simulink model "autotun2_1stor_mod"  (R2025b)
settings: Solver=ode4  StartTime=0.0  StopTime=50  FixedStep=Tm  RelTol=1e-3
values from neighbouring files (symbols this model uses):
  Delay = 0.005    [twodo_par1.m]
  Tm = St    (= 0.001)    [twodo_par1.m]
libraries: fuzblock x2
settings Model: ExtModeTrigMode=oneshot  ExtModeArmWhenConnect=off  Creator=rel  LastModifiedBy=labrobm
settings DataIOCC: SaveFormat=Array  SignalLoggingSaveFormat=ModelDataLogs  ReturnWorkspaceOutputs=off  SignalLoggingName=sigsOut
settings OptimizationCC: BlockReduction=off  BooleanDataType=off
settings DebuggingCC: SaveWithParameterizedLinksMsg=none  UnderspecifiedInitializationDetection=Classic  MergeDetectMultiDrivingBlocksExec=none  SignalResolutionControl=TryResolveAllWithWarning  MultiTaskDSMMsg=warning  MultiTaskCondExecSysMsg=none  UnconnectedInputMsg=warning  UnconnectedOutputMsg=warning  UnconnectedLineMsg=warning
settings HardwareCC: ProdBitPerPointer=32.0  ProdBitPerSizeT=32.0  ProdBitPerPtrDiffT=32.0  ProdLargestAtomicFloat=None  ProdIntDivRoundTo=Undefined  ProdEndianess=Unspecified  ProdWordSize=32.0  ProdHWDeviceType=32-bit Generic  TargetUnknown=on
settings ModelReferenceCC: PropagateSignalLabelsOutOfModel=off
settings GRTTargetCC: CombineOutputUpdateFcns=off  GRTInterface=on
settings ConfigComp: CovMetricSettings=dw  CovSaveCumulativeToWorkspaceVar=on  CovSaveSingleToWorkspaceVar=on

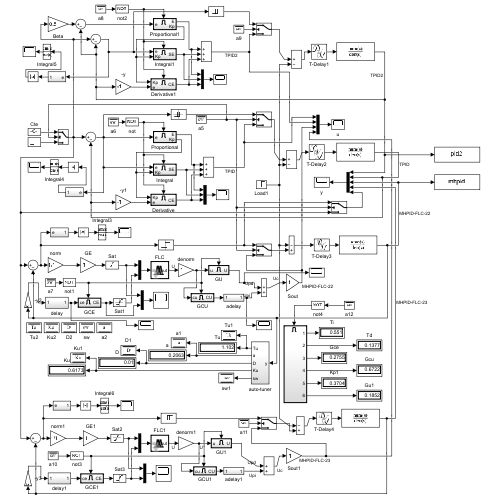
[thumbnail: Simulink's stored preview of the top-level diagram]
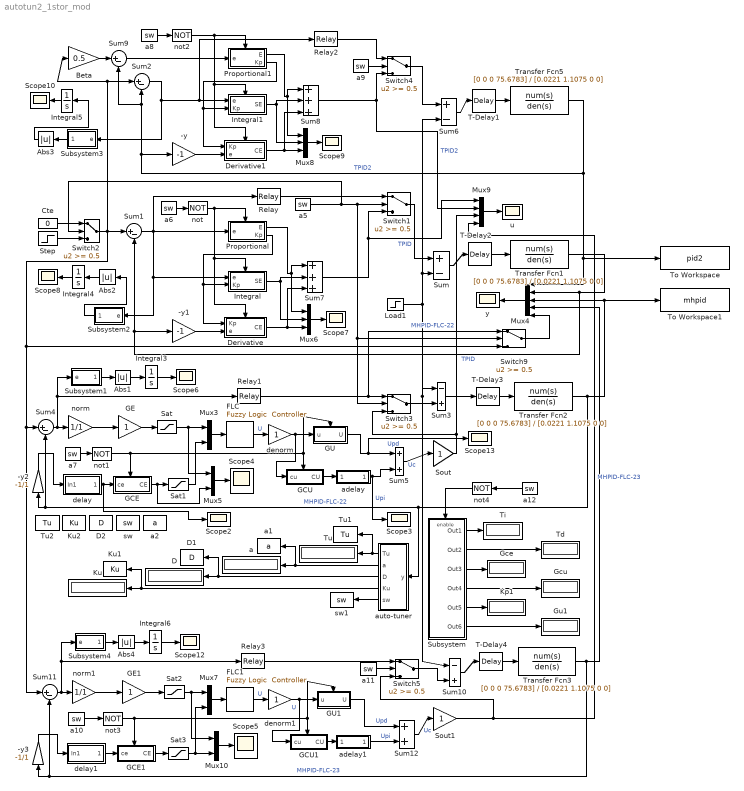
== system autotun2_1stor_mod ==
  -y : Gain  Gain=-1  SaturateOnIntegerOverflow=on  OutDataTypeStr=Inherit: Same as input  ParamDataTypeStr=Inherit: Same as input
  -y1 : Gain  Gain=-1  SaturateOnIntegerOverflow=on  OutDataTypeStr=Inherit: Same as input  ParamDataTypeStr=Inherit: Same as input
  -y2 : Gain  Gain=-1/1  SaturateOnIntegerOverflow=on  OutDataTypeStr=Inherit: Same as input  ParamDataTypeStr=Inherit: Same as input
  -y3 : Gain  Gain=-1/1  SaturateOnIntegerOverflow=on  OutDataTypeStr=Inherit: Same as input  ParamDataTypeStr=Inherit: Same as input
  Abs{1..4} (4 alike) : Abs
  Beta : Gain  Gain=0.5  SaturateOnIntegerOverflow=on  OutDataTypeStr=Inherit: Same as input  ParamDataTypeStr=Inherit: Same as input
  Cte : Constant  Value=0
  D : Display
  D1 : DataStoreWrite  DataStoreName=D  IndexOptions=Index vector (dialog)  Indices=1  OutputSizes=1
  D2 : DataStoreMemory  DataStoreName=D  ShowAdditionalParam=off
  Derivative : Subsystem  TreatAsAtomicUnit=on
  Derivative1 : Subsystem  TreatAsAtomicUnit=on
  FLC : fuzblock/Fuzzy Logic  Controller  FIS=stfc22  OutputSampleNumber=101  DataType=double  UseLookupTable=off  NumBreakpoints=10  FuzzifiedInputs=off  RuleFiringStrengths=off  RuleOutputs=off  AggregatedOutputs=off  SimulateUsing=Interpreted execution  OutOfRangeInputValueMessage=warning  NoRuleFiredMessage=warning  EmptyOutputFuzzySetMessage=warning
  FLC1 : fuzblock/Fuzzy Logic  Controller  FIS=stfc23  OutputSampleNumber=101  DataType=double  UseLookupTable=off  NumBreakpoints=10  FuzzifiedInputs=off  RuleFiringStrengths=off  RuleOutputs=off  AggregatedOutputs=off  SimulateUsing=Interpreted execution  OutOfRangeInputValueMessage=warning  NoRuleFiredMessage=warning  EmptyOutputFuzzySetMessage=warning
  GCE : Subsystem  TreatAsAtomicUnit=on
  GCE1 : Subsystem  TreatAsAtomicUnit=on
  GCU : Subsystem  TreatAsAtomicUnit=on
  GCU1 : Subsystem  TreatAsAtomicUnit=on
  GE : Gain  SaturateOnIntegerOverflow=on  OutDataTypeStr=Inherit: Same as input  ParamDataTypeStr=Inherit: Same as input
  GE1 : Gain  SaturateOnIntegerOverflow=on  OutDataTypeStr=Inherit: Same as input  ParamDataTypeStr=Inherit: Same as input
  GU : Subsystem  TreatAsAtomicUnit=on
  GU1 : Subsystem  TreatAsAtomicUnit=on
  Gce : Display
  Gcu : Display
  Gu1 : Display
  Integral : Subsystem  TreatAsAtomicUnit=on
  Integral1 : Subsystem  TreatAsAtomicUnit=on
  Integral{3..6} (4 alike) : TransferFcn  Denominator=[1 0]
  Kp1 : Display
  Ku : Display
  Ku1 : DataStoreWrite  DataStoreName=Ku  IndexOptions=Index vector (dialog)  Indices=1  OutputSizes=1
  Ku2 : DataStoreMemory  DataStoreName=Ku  ShowAdditionalParam=off
  Load1 : Step  Time=40  SampleTime=0
  Mux{3,5,7,10} (4 alike) : Mux  Inputs=2
  Mux4 : Mux  Inputs=5
  Mux6 : Mux  Inputs=3
  Mux8 : Mux  Inputs=3
  Mux9 : Mux
  Proportional : Subsystem  TreatAsAtomicUnit=on
  Proportional1 : Subsystem  TreatAsAtomicUnit=on
  Relay{,1..3} (4 alike) : Relay  OnOutputValue=0.1  OffOutputValue=-0.1
  Sat{,1..3} (4 alike) : Saturate  UpperLimit=1  LowerLimit=-1
  Scope{2..10,12..13} (11 alike) : Scope
      Scope10 settings: TimeSpan=40  ActiveDisplayYMinimum=0  ActiveDisplayYMaximum=1.5
      Scope12 settings: TimeSpan=40  ActiveDisplayYMinimum=0  ActiveDisplayYMaximum=1.73154
      Scope13 settings: TimeSpan=50  ActiveDisplayYMinimum=-0.01  ActiveDisplayYMaximum=0.05
      Scope2 settings: TimeSpan=50  ActiveDisplayYMinimum=-0.02  ActiveDisplayYMaximum=0.01
      Scope3 settings: TimeSpan=50  ActiveDisplayYMinimum=-0.90801012374905665  ActiveDisplayYMaximum=1.7443936739549131
      Scope4 settings: TimeSpan=50  ActiveDisplayYMinimum=-1  ActiveDisplayYMaximum=1
      Scope5 settings: TimeSpan=40  ActiveDisplayYMinimum=-1  ActiveDisplayYMaximum=1
      Scope6 settings: TimeSpan=40  ActiveDisplayYMinimum=0  ActiveDisplayYMaximum=2
      Scope7 settings: TimeSpan=40  ActiveDisplayYMinimum=-50  ActiveDisplayYMaximum=150
      Scope8 settings: TimeSpan=40  ActiveDisplayYMinimum=0  ActiveDisplayYMaximum=1.77181
      Scope9 settings: TimeSpan=50  ActiveDisplayYMinimum=-2.71141  ActiveDisplayYMaximum=4
  Sout : Gain  SaturateOnIntegerOverflow=on  OutDataTypeStr=Inherit: Same as input  ParamDataTypeStr=Inherit: Same as input
  Sout1 : Gain  SaturateOnIntegerOverflow=on  OutDataTypeStr=Inherit: Same as input  ParamDataTypeStr=Inherit: Same as input
  Step : Step  Time=30  SampleTime=0
  Subsystem : Subsystem  TreatAsAtomicUnit=on
  Subsystem1 : Subsystem
  Subsystem2 : Subsystem
  Subsystem3 : Subsystem
  Subsystem4 : Subsystem
  Sum{,1..2,4,6,9,11} (7 alike) : Sum  Inputs=|+-  InputSameDT=on  SaturateOnIntegerOverflow=on  OutDataTypeStr=Inherit: Same as first input
  Sum10 : Sum  Inputs=|-+  InputSameDT=on  SaturateOnIntegerOverflow=on  OutDataTypeStr=Inherit: Same as first input
  Sum12 : Sum  Inputs=|++  InputSameDT=on  SaturateOnIntegerOverflow=on  OutDataTypeStr=Inherit: Same as first input
  Sum3 : Sum  Inputs=|-+  InputSameDT=on  SaturateOnIntegerOverflow=on  OutDataTypeStr=Inherit: Same as first input
  Sum5 : Sum  Inputs=|++  InputSameDT=on  SaturateOnIntegerOverflow=on  OutDataTypeStr=Inherit: Same as first input
  Sum7 : Sum  Inputs=|+++  InputSameDT=on  SaturateOnIntegerOverflow=on  OutDataTypeStr=Inherit: Same as first input
  Sum8 : Sum  Inputs=|+++  InputSameDT=on  SaturateOnIntegerOverflow=on  OutDataTypeStr=Inherit: Same as first input
  Switch{1..5,9} (6 alike) : Switch  Threshold=0.5
  T-Delay{1..4} (4 alike) : TransportDelay  DelayTime=Delay
  Td : Display
  Ti : Display
  To Workspace : ToWorkspace  VariableName=pid2  SaveFormat=Timeseries  SampleTime=-1
  To Workspace1 : ToWorkspace  VariableName=mhpid  SaveFormat=Timeseries  SampleTime=-1
  Transfer Fcn{1..3,5} (4 alike) : TransferFcn  Numerator=[0 0 0 75.6783]  Denominator=[0.0221 1.1075 0 0]
  Tu : Display
  Tu1 : DataStoreWrite  DataStoreName=Tu  IndexOptions=Index vector (dialog)  Indices=1  OutputSizes=1
  Tu2 : DataStoreMemory  DataStoreName=Tu  InitialValue=1  ShowAdditionalParam=off
  a : Display
  a1 : DataStoreWrite  DataStoreName=a  IndexOptions=Index vector (dialog)  Indices=1  OutputSizes=1
  a{5..12} (8 alike) : DataStoreRead  DataStoreName=sw  SampleTime=0  IndexOptions=Index vector (dialog)  Indices=1  OutputSizes=1
  a2 : DataStoreMemory  DataStoreName=a  ShowAdditionalParam=off
  adelay : Subsystem
  adelay1 : Subsystem
  auto-tuner : Subsystem
  delay : Subsystem
  delay1 : Subsystem
  denorm : Gain  SaturateOnIntegerOverflow=on  OutDataTypeStr=Inherit: Same as input  ParamDataTypeStr=Inherit: Same as input
  denorm1 : Gain  SaturateOnIntegerOverflow=on  OutDataTypeStr=Inherit: Same as input  ParamDataTypeStr=Inherit: Same as input
  norm : Gain  Gain=1/1  SaturateOnIntegerOverflow=on  OutDataTypeStr=Inherit: Same as input  ParamDataTypeStr=Inherit: Same as input
  norm1 : Gain  Gain=1/1  SaturateOnIntegerOverflow=on  OutDataTypeStr=Inherit: Same as input  ParamDataTypeStr=Inherit: Same as input
  not{,1..4} (5 alike) : Logic  Operator=NOT
  sw : DataStoreMemory  DataStoreName=sw  ShowAdditionalParam=off
  sw1 : DataStoreWrite  DataStoreName=sw  IndexOptions=Index vector (dialog)  Indices=1  OutputSizes=1
  u : Scope
      settings: TimeSpan=50  ActiveDisplayYMinimum=-2.2972256680576972  ActiveDisplayYMaximum=2.8129712907117121
  y : Scope
      settings: TimeSpan=50  ActiveDisplayYMinimum=-2.7790982522608521  ActiveDisplayYMaximum=3.0464036991149257  DataLoggingVariableName=G3
  wires:
  T-Delay2/1 -> Transfer Fcn1/1
  Mux4/1 -> y/1
  Mux3/1 -> FLC/1
  T-Delay3/1 -> Transfer Fcn2/1
  Step/1 -> Switch2/3
  Cte/1 -> Switch2/1
  Transfer Fcn2/1 -> auto-tuner/1(y), Sum4/2, -y2/1, To Workspace1/1, Mux4/3  "MHPID-FLC-22"
  Sum1/1 -> Proportional/1(e), Integral/1(e), Subsystem2/1(e), Relay/1
  Sum5/1 -> Sout/1  "Uc"
  a6/1 -> not/1
  not/1 -> Proportional/Enable, Integral/Enable, Derivative/Enable
  Proportional/2(Kp) -> Derivative/1(Kp), Integral/2(Kp)
  a7/1 -> not1/1
  Mux5/1 -> Scope4/1
  not1/1 -> GCE/Enable, GCU/Enable, GU/Enable
  Switch2/1 -> Switch9/3, Sum4/1, Sum11/1, Sum1/1, Sum2/1, Beta/1
  Load1/1 -> Sum6/2, Sum/2, Sum3/1, Sum10/1
  auto-tuner/1(Tu) -> Tu/1, Tu1/1
  auto-tuner/2(a) -> a/1, a1/1
  auto-tuner/3(D) -> D/1, D1/1
  auto-tuner/4(Ku) -> Ku/1, Ku1/1
  auto-tuner/5(sw) -> sw1/1
  Subsystem1/1(Out1) -> Abs1/1
  Abs1/1 -> Integral3/1
  Integral3/1 -> Scope6/1
  Integral4/1 -> Scope8/1
  Abs2/1 -> Integral4/1
  Subsystem2/1(Out1) -> Abs2/1
  Proportional1/2(Kp) -> Derivative1/1(Kp), Integral1/2(Kp)
  a8/1 -> not2/1
  not2/1 -> Proportional1/Enable, Derivative1/Enable, Integral1/Enable
  T-Delay1/1 -> Transfer Fcn5/1
  Beta/1 -> Sum9/1
  Sum2/1 -> Integral1/1(e), Relay2/1, Subsystem3/1(e)
  Sum9/1 -> Proportional1/1(e)
  a5/1 -> Switch3/2, Switch9/2, Switch1/2, Switch2/2
  Mux6/1 -> Scope7/1
  Derivative/1(CE) -> Sum7/3, Mux6/3
  Mux8/1 -> Scope9/1
  Derivative1/1(CE) -> Sum8/3, Mux8/3
  Integral1/1(SE) -> Sum8/2, Mux8/2
  Proportional1/1(E) -> Sum8/1, Mux8/1
  Integral/1(SE) -> Sum7/2, Mux6/2
  Proportional/1(E) -> Sum7/1, Mux6/1
  a9/1 -> Switch4/2
  Relay2/1 -> Switch4/1
  Switch4/1 -> Sum6/1
  Sum4/1 -> Subsystem1/1(e), Relay1/1, norm/1
  Relay/1 -> Switch1/1
  Relay1/1 -> Switch3/1, Switch9/1
  Integral5/1 -> Scope10/1
  Subsystem3/1(Out1) -> Abs3/1
  Abs3/1 -> Integral5/1
  Mux9/1 -> u/1
  Sum6/1 -> T-Delay1/1
  Sum/1 -> T-Delay2/1
  Sum3/1 -> T-Delay3/1
  Sum8/1 -> Switch4/3, Mux9/2  "TPID2"
  Mux7/1 -> FLC1/1
  adelay1/1(Out1) -> Sum12/2  "Upi"
  T-Delay4/1 -> Transfer Fcn3/1
  Sum12/1 -> Sout1/1  "Uc"
  GCU1/1(CU) -> adelay1/1(In1)
  a10/1 -> not3/1
  delay1/1(Out1) -> GCE1/1(ce)
  Mux10/1 -> Scope5/1
  not3/1 -> GCE1/Enable, GCU1/Enable, GU1/Enable
  FLC1/1 -> denorm1/1  "U"
  GU1/1(U) -> Sum12/1  "Upd"
  Subsystem4/1(Out1) -> Abs4/1
  Abs4/1 -> Integral6/1
  Integral6/1 -> Scope12/1
  Sum11/1 -> Subsystem4/1(e), Relay3/1, norm1/1
  Switch5/1 -> Sum10/2
  Sum10/1 -> T-Delay4/1
  GCE1/1(CE) -> Sat3/1
  Sat3/1 -> Mux7/2, Mux10/2
  GE1/1 -> Sat2/1
  Sat2/1 -> Mux7/1, Mux10/1
  Relay3/1 -> Switch5/1
  a11/1 -> Switch5/2
  Transfer Fcn3/1 -> Mux4/4, Sum11/2, -y3/1  "MHPID-FLC-23"
  norm/1 -> GE/1
  Subsystem/1(Out1) -> Ti/1
  Subsystem/3(Out3) -> Gce/1
  Subsystem/5(Out5) -> Kp1/1
  a12/1 -> not4/1
  not4/1 -> Subsystem/Enable
  Subsystem/2(Out2) -> Td/1
  Subsystem/6(Out6) -> Gu1/1
  Transfer Fcn5/1 -> Sum2/2, Sum9/2, -y/1, To Workspace/1, Mux4/1  "TPID2"
  Transfer Fcn1/1 -> Sum1/2, -y1/1, Mux4/2  "TPID"
  Sout1/1 -> Switch5/3, Mux9/4  "MHPID-FLC-23"
  Switch1/1 -> Sum/1
  Sum7/1 -> Switch1/3, Mux9/1  "TPID"
  Subsystem/4(Out4) -> Gcu/1
  Sat/1 -> Mux3/1, Mux5/1
  GE/1 -> Sat/1
  Sat1/1 -> Mux3/2
  GCE/1(CE) -> Sat1/1, Mux5/2
  Switch3/1 -> Sum3/2
  Sout/1 -> Switch3/3, Mux9/3  "MHPID-FLC-22"
  delay/1(Out1) -> GCE/1(ce), Scope2/1
  GCU/1(CU) -> adelay/1(In1)
  adelay/1(Out1) -> Sum5/2, Scope3/1  "Upi"
  GU/1(U) -> Sum5/1, Scope13/1  "Upd"
  -y/1 -> Derivative1/2(e)
  -y1/1 -> Derivative/2(e)
  -y2/1 -> delay/1(In1)
  norm1/1 -> GE1/1
  -y3/1 -> delay1/1(In1)
  denorm/1 -> GU/1(u), GCU/1(cu)
  FLC/1 -> denorm/1  "U"
  denorm1/1 -> GCU1/1(cu), GU1/1(u)  "U"
  Switch9/1 -> Mux4/5

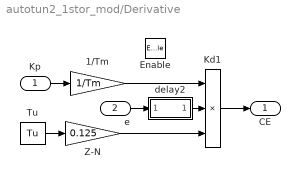
== system autotun2_1stor_mod/Derivative ==
  Kp : Inport
  e : Inport  Port=2
  Enable : EnablePort
  1/Tm : Gain  Gain=1/Tm  SaturateOnIntegerOverflow=on  OutDataTypeStr=Inherit: Same as input  ParamDataTypeStr=Inherit: Same as input
  Kd1 : Product  Inputs=3  InputSameDT=on  SaturateOnIntegerOverflow=on  OutDataTypeStr=Inherit: Same as first input
  Tu : DataStoreRead  DataStoreName=Tu  SampleTime=0  IndexOptions=Index vector (dialog)  Indices=1  OutputSizes=1
  Z-N : Gain  Gain=0.125  SaturateOnIntegerOverflow=on  OutDataTypeStr=Inherit: Same as input  ParamDataTypeStr=Inherit: Same as input
  delay2 : Subsystem
  CE : Outport
  wires:
  e/1 -> delay2/1(In1)
  Kd1/1 -> CE/1
  Tu/1 -> Z-N/1
  Z-N/1 -> Kd1/3
  Kp/1 -> 1/Tm/1
  1/Tm/1 -> Kd1/1
  delay2/1(Out1) -> Kd1/2

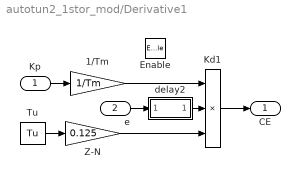
== system autotun2_1stor_mod/Derivative1 ==
  Kp : Inport
  e : Inport  Port=2
  Enable : EnablePort
  1/Tm : Gain  Gain=1/Tm  SaturateOnIntegerOverflow=on  OutDataTypeStr=Inherit: Same as input  ParamDataTypeStr=Inherit: Same as input
  Kd1 : Product  Inputs=3  InputSameDT=on  SaturateOnIntegerOverflow=on  OutDataTypeStr=Inherit: Same as first input
  Tu : DataStoreRead  DataStoreName=Tu  SampleTime=0  IndexOptions=Index vector (dialog)  Indices=1  OutputSizes=1
  Z-N : Gain  Gain=0.125  SaturateOnIntegerOverflow=on  OutDataTypeStr=Inherit: Same as input  ParamDataTypeStr=Inherit: Same as input
  delay2 : Subsystem
  CE : Outport
  wires:
  e/1 -> delay2/1(In1)
  Kd1/1 -> CE/1
  Tu/1 -> Z-N/1
  Z-N/1 -> Kd1/3
  Kp/1 -> 1/Tm/1
  1/Tm/1 -> Kd1/1
  delay2/1(Out1) -> Kd1/2

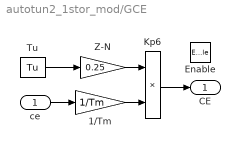
== system autotun2_1stor_mod/GCE ==
  ce : Inport
  Enable : EnablePort
  1/Tm : Gain  Gain=1/Tm  SaturateOnIntegerOverflow=on  OutDataTypeStr=Inherit: Same as input  ParamDataTypeStr=Inherit: Same as input
  Kp6 : Product  InputSameDT=on  SaturateOnIntegerOverflow=on  OutDataTypeStr=Inherit: Same as first input
  Tu : DataStoreRead  DataStoreName=Tu  SampleTime=0  IndexOptions=Index vector (dialog)  Indices=1  OutputSizes=1
  Z-N : Gain  Gain=0.25  SaturateOnIntegerOverflow=on  OutDataTypeStr=Inherit: Same as input  ParamDataTypeStr=Inherit: Same as input
  CE : Outport
  wires:
  Kp6/1 -> CE/1
  Tu/1 -> Z-N/1
  Z-N/1 -> Kp6/1
  ce/1 -> 1/Tm/1
  1/Tm/1 -> Kp6/2

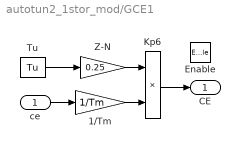
== system autotun2_1stor_mod/GCE1 ==
  ce : Inport
  Enable : EnablePort
  1/Tm : Gain  Gain=1/Tm  SaturateOnIntegerOverflow=on  OutDataTypeStr=Inherit: Same as input  ParamDataTypeStr=Inherit: Same as input
  Kp6 : Product  InputSameDT=on  SaturateOnIntegerOverflow=on  OutDataTypeStr=Inherit: Same as first input
  Tu : DataStoreRead  DataStoreName=Tu  SampleTime=0  IndexOptions=Index vector (dialog)  Indices=1  OutputSizes=1
  Z-N : Gain  Gain=0.25  SaturateOnIntegerOverflow=on  OutDataTypeStr=Inherit: Same as input  ParamDataTypeStr=Inherit: Same as input
  CE : Outport
  wires:
  Kp6/1 -> CE/1
  Tu/1 -> Z-N/1
  Z-N/1 -> Kp6/1
  ce/1 -> 1/Tm/1
  1/Tm/1 -> Kp6/2

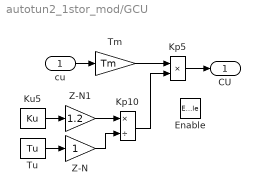
== system autotun2_1stor_mod/GCU ==
  cu : Inport
  Enable : EnablePort
  Kp10 : Product  Inputs=*/  InputSameDT=on  SaturateOnIntegerOverflow=on  OutDataTypeStr=Inherit: Same as first input
  Kp5 : Product  InputSameDT=on  SaturateOnIntegerOverflow=on  OutDataTypeStr=Inherit: Same as first input
  Ku5 : DataStoreRead  DataStoreName=Ku  SampleTime=0  IndexOptions=Index vector (dialog)  Indices=1  OutputSizes=1
  Tm : Gain  Gain=Tm  SaturateOnIntegerOverflow=on  OutDataTypeStr=Inherit: Same as input  ParamDataTypeStr=Inherit: Same as input
  Tu : DataStoreRead  DataStoreName=Tu  SampleTime=0  IndexOptions=Index vector (dialog)  Indices=1  OutputSizes=1
  Z-N : Gain  SaturateOnIntegerOverflow=on  OutDataTypeStr=Inherit: Same as input  ParamDataTypeStr=Inherit: Same as input
  Z-N1 : Gain  Gain=1.2  SaturateOnIntegerOverflow=on  OutDataTypeStr=Inherit: Same as input  ParamDataTypeStr=Inherit: Same as input
  CU : Outport
  wires:
  Tu/1 -> Z-N/1
  Z-N/1 -> Kp10/2
  Ku5/1 -> Z-N1/1
  Kp5/1 -> CU/1
  Z-N1/1 -> Kp10/1
  cu/1 -> Tm/1
  Tm/1 -> Kp5/1
  Kp10/1 -> Kp5/2

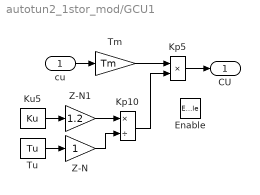
== system autotun2_1stor_mod/GCU1 ==
  cu : Inport
  Enable : EnablePort
  Kp10 : Product  Inputs=*/  InputSameDT=on  SaturateOnIntegerOverflow=on  OutDataTypeStr=Inherit: Same as first input
  Kp5 : Product  InputSameDT=on  SaturateOnIntegerOverflow=on  OutDataTypeStr=Inherit: Same as first input
  Ku5 : DataStoreRead  DataStoreName=Ku  SampleTime=0  IndexOptions=Index vector (dialog)  Indices=1  OutputSizes=1
  Tm : Gain  Gain=Tm  SaturateOnIntegerOverflow=on  OutDataTypeStr=Inherit: Same as input  ParamDataTypeStr=Inherit: Same as input
  Tu : DataStoreRead  DataStoreName=Tu  SampleTime=0  IndexOptions=Index vector (dialog)  Indices=1  OutputSizes=1
  Z-N : Gain  SaturateOnIntegerOverflow=on  OutDataTypeStr=Inherit: Same as input  ParamDataTypeStr=Inherit: Same as input
  Z-N1 : Gain  Gain=1.2  SaturateOnIntegerOverflow=on  OutDataTypeStr=Inherit: Same as input  ParamDataTypeStr=Inherit: Same as input
  CU : Outport
  wires:
  Tu/1 -> Z-N/1
  Z-N/1 -> Kp10/2
  Ku5/1 -> Z-N1/1
  Kp5/1 -> CU/1
  Z-N1/1 -> Kp10/1
  cu/1 -> Tm/1
  Tm/1 -> Kp5/1
  Kp10/1 -> Kp5/2

== system autotun2_1stor_mod/GU ==
  u : Inport
  Enable : EnablePort
  Kp7 : Product  InputSameDT=on  SaturateOnIntegerOverflow=on  OutDataTypeStr=Inherit: Same as first input
  Ku5 : DataStoreRead  DataStoreName=Ku  SampleTime=0  IndexOptions=Index vector (dialog)  Indices=1  OutputSizes=1
  Z-N1 : Gain  Gain=0.3  SaturateOnIntegerOverflow=on  OutDataTypeStr=Inherit: Same as input  ParamDataTypeStr=Inherit: Same as input
  U : Outport
  wires:
  Kp7/1 -> U/1
  u/1 -> Kp7/2
  Ku5/1 -> Z-N1/1
  Z-N1/1 -> Kp7/1

== system autotun2_1stor_mod/GU1 ==
  u : Inport
  Enable : EnablePort
  Kp7 : Product  InputSameDT=on  SaturateOnIntegerOverflow=on  OutDataTypeStr=Inherit: Same as first input
  Ku5 : DataStoreRead  DataStoreName=Ku  SampleTime=0  IndexOptions=Index vector (dialog)  Indices=1  OutputSizes=1
  Z-N1 : Gain  Gain=0.3  SaturateOnIntegerOverflow=on  OutDataTypeStr=Inherit: Same as input  ParamDataTypeStr=Inherit: Same as input
  U : Outport
  wires:
  Kp7/1 -> U/1
  u/1 -> Kp7/2
  Ku5/1 -> Z-N1/1
  Z-N1/1 -> Kp7/1

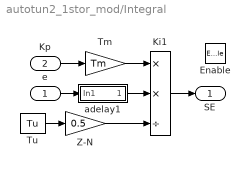
== system autotun2_1stor_mod/Integral ==
  e : Inport
  Kp : Inport  Port=2
  Enable : EnablePort
  Ki1 : Product  Inputs=**/  InputSameDT=on  SaturateOnIntegerOverflow=on  OutDataTypeStr=Inherit: Same as first input
  Tm : Gain  Gain=Tm  SaturateOnIntegerOverflow=on  OutDataTypeStr=Inherit: Same as input  ParamDataTypeStr=Inherit: Same as input
  Tu : DataStoreRead  DataStoreName=Tu  SampleTime=0  IndexOptions=Index vector (dialog)  Indices=1  OutputSizes=1
  Z-N : Gain  Gain=0.5  SaturateOnIntegerOverflow=on  OutDataTypeStr=Inherit: Same as input  ParamDataTypeStr=Inherit: Same as input
  adelay1 : Subsystem
  SE : Outport
  wires:
  adelay1/1(Out1) -> Ki1/2
  Z-N/1 -> Ki1/3
  e/1 -> adelay1/1(In1)
  Ki1/1 -> SE/1
  Tu/1 -> Z-N/1
  Kp/1 -> Tm/1
  Tm/1 -> Ki1/1

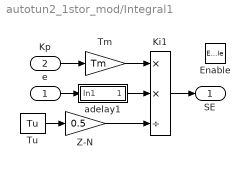
== system autotun2_1stor_mod/Integral1 ==
  e : Inport
  Kp : Inport  Port=2
  Enable : EnablePort
  Ki1 : Product  Inputs=**/  InputSameDT=on  SaturateOnIntegerOverflow=on  OutDataTypeStr=Inherit: Same as first input
  Tm : Gain  Gain=Tm  SaturateOnIntegerOverflow=on  OutDataTypeStr=Inherit: Same as input  ParamDataTypeStr=Inherit: Same as input
  Tu : DataStoreRead  DataStoreName=Tu  SampleTime=0  IndexOptions=Index vector (dialog)  Indices=1  OutputSizes=1
  Z-N : Gain  Gain=0.5  SaturateOnIntegerOverflow=on  OutDataTypeStr=Inherit: Same as input  ParamDataTypeStr=Inherit: Same as input
  adelay1 : Subsystem
  SE : Outport
  wires:
  adelay1/1(Out1) -> Ki1/2
  Z-N/1 -> Ki1/3
  e/1 -> adelay1/1(In1)
  Ki1/1 -> SE/1
  Tu/1 -> Z-N/1
  Kp/1 -> Tm/1
  Tm/1 -> Ki1/1

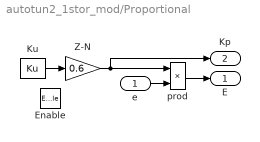
== system autotun2_1stor_mod/Proportional ==
  e : Inport
  Enable : EnablePort
  Ku : DataStoreRead  DataStoreName=Ku  SampleTime=0  IndexOptions=Index vector (dialog)  Indices=1  OutputSizes=1
  Z-N : Gain  Gain=0.6  SaturateOnIntegerOverflow=on  OutDataTypeStr=Inherit: Same as input  ParamDataTypeStr=Inherit: Same as input
  prod : Product  InputSameDT=on  SaturateOnIntegerOverflow=on  OutDataTypeStr=Inherit: Same as first input
  E : Outport
  Kp : Outport  Port=2
  wires:
  Ku/1 -> Z-N/1
  prod/1 -> E/1
  e/1 -> prod/2
  Z-N/1 -> Kp/1, prod/1

== system autotun2_1stor_mod/Proportional1 ==
  e : Inport
  Enable : EnablePort
  Ku : DataStoreRead  DataStoreName=Ku  SampleTime=0  IndexOptions=Index vector (dialog)  Indices=1  OutputSizes=1
  Z-N : Gain  Gain=0.6  SaturateOnIntegerOverflow=on  OutDataTypeStr=Inherit: Same as input  ParamDataTypeStr=Inherit: Same as input
  prod : Product  InputSameDT=on  SaturateOnIntegerOverflow=on  OutDataTypeStr=Inherit: Same as first input
  E : Outport
  Kp : Outport  Port=2
  wires:
  prod/1 -> E/1
  e/1 -> prod/2
  Z-N/1 -> prod/1, Kp/1
  Ku/1 -> Z-N/1

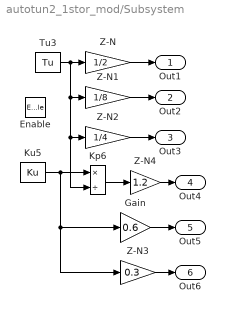
== system autotun2_1stor_mod/Subsystem ==
  Enable : EnablePort
  Gain : Gain  Gain=0.6  SaturateOnIntegerOverflow=on  OutDataTypeStr=Inherit: Same as input  ParamDataTypeStr=Inherit: Same as input
  Kp6 : Product  Inputs=*/  InputSameDT=on  SaturateOnIntegerOverflow=on  OutDataTypeStr=Inherit: Same as first input
  Ku5 : DataStoreRead  DataStoreName=Ku  SampleTime=0  IndexOptions=Index vector (dialog)  Indices=1  OutputSizes=1
  Tu3 : DataStoreRead  DataStoreName=Tu  SampleTime=0  IndexOptions=Index vector (dialog)  Indices=1  OutputSizes=1
  Z-N : Gain  Gain=1/2  SaturateOnIntegerOverflow=on  OutDataTypeStr=Inherit: Same as input  ParamDataTypeStr=Inherit: Same as input
  Z-N1 : Gain  Gain=1/8  SaturateOnIntegerOverflow=on  OutDataTypeStr=Inherit: Same as input  ParamDataTypeStr=Inherit: Same as input
  Z-N2 : Gain  Gain=1/4  SaturateOnIntegerOverflow=on  OutDataTypeStr=Inherit: Same as input  ParamDataTypeStr=Inherit: Same as input
  Z-N3 : Gain  Gain=0.3  SaturateOnIntegerOverflow=on  OutDataTypeStr=Inherit: Same as input  ParamDataTypeStr=Inherit: Same as input
  Z-N4 : Gain  Gain=1.2  SaturateOnIntegerOverflow=on  OutDataTypeStr=Inherit: Same as input  ParamDataTypeStr=Inherit: Same as input
  Out1 : Outport
  Out2 : Outport  Port=2
  Out3 : Outport  Port=3
  Out4 : Outport  Port=4
  Out5 : Outport  Port=5
  Out6 : Outport  Port=6
  wires:
  Tu3/1 -> Z-N/1, Z-N1/1, Z-N2/1, Kp6/2
  Kp6/1 -> Z-N4/1
  Z-N/1 -> Out1/1
  Z-N1/1 -> Out2/1
  Z-N2/1 -> Out3/1
  Z-N4/1 -> Out4/1
  Z-N3/1 -> Out6/1
  Gain/1 -> Out5/1
  Ku5/1 -> Kp6/1, Gain/1, Z-N3/1

== system autotun2_1stor_mod/Subsystem1 ==
  e : Inport
  Clock1 : Clock
  Equal3 : RelationalOperator  Operator=<
  Switch4 : Switch  Threshold=0.5
  zero : Constant  Value=0
  zero1 : Constant  Value=20
  Out1 : Outport
  wires:
  Clock1/1 -> Equal3/1
  zero1/1 -> Equal3/2
  Switch4/1 -> Out1/1
  e/1 -> Switch4/3
  zero/1 -> Switch4/1
  Equal3/1 -> Switch4/2

== system autotun2_1stor_mod/Subsystem2 ==
  e : Inport
  Clock1 : Clock
  Equal3 : RelationalOperator  Operator=<
  Switch4 : Switch  Threshold=0.5
  zero : Constant  Value=0
  zero1 : Constant  Value=20
  Out1 : Outport
  wires:
  Clock1/1 -> Equal3/1
  zero1/1 -> Equal3/2
  Switch4/1 -> Out1/1
  e/1 -> Switch4/3
  zero/1 -> Switch4/1
  Equal3/1 -> Switch4/2

== system autotun2_1stor_mod/Subsystem3 ==
  e : Inport
  Clock1 : Clock
  Equal3 : RelationalOperator  Operator=<
  Switch4 : Switch  Threshold=0.5
  zero : Constant  Value=0
  zero1 : Constant  Value=20
  Out1 : Outport
  wires:
  Clock1/1 -> Equal3/1
  zero1/1 -> Equal3/2
  Switch4/1 -> Out1/1
  e/1 -> Switch4/3
  zero/1 -> Switch4/1
  Equal3/1 -> Switch4/2

== system autotun2_1stor_mod/Subsystem4 ==
  e : Inport
  Clock1 : Clock
  Equal3 : RelationalOperator  Operator=<
  Switch4 : Switch  Threshold=0.5
  zero : Constant  Value=0
  zero1 : Constant  Value=20
  Out1 : Outport
  wires:
  Clock1/1 -> Equal3/1
  zero1/1 -> Equal3/2
  Switch4/1 -> Out1/1
  e/1 -> Switch4/3
  zero/1 -> Switch4/1
  Equal3/1 -> Switch4/2

== system autotun2_1stor_mod/adelay ==
  In1 : Inport
  Sum9 : Sum  Inputs=|++  InputSameDT=on  SaturateOnIntegerOverflow=on  OutDataTypeStr=Inherit: Same as first input
  Unit Delay6 : UnitDelay  SampleTime=Tm
  Out1 : Outport
  wires:
  In1/1 -> Sum9/1
  Unit Delay6/1 -> Sum9/2
  Sum9/1 -> Out1/1, Unit Delay6/1

== system autotun2_1stor_mod/adelay1 ==
  In1 : Inport
  Sum9 : Sum  Inputs=|++  InputSameDT=on  SaturateOnIntegerOverflow=on  OutDataTypeStr=Inherit: Same as first input
  Unit Delay6 : UnitDelay  SampleTime=Tm
  Out1 : Outport
  wires:
  In1/1 -> Sum9/1
  Unit Delay6/1 -> Sum9/2
  Sum9/1 -> Out1/1, Unit Delay6/1

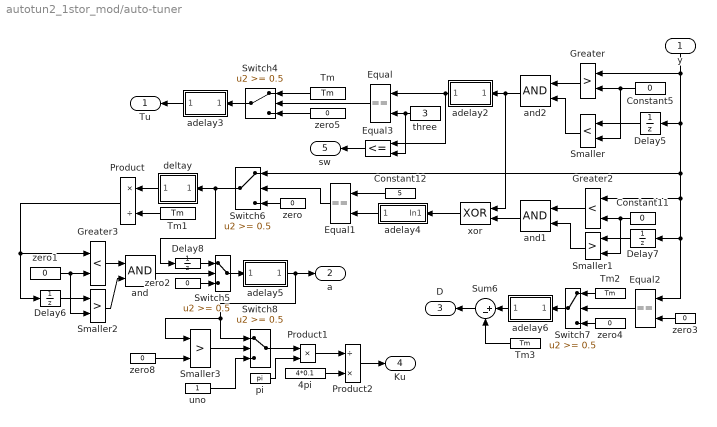
== system autotun2_1stor_mod/auto-tuner ==
  y : Inport
  4pi : Constant  Value=4*0.1
  Constant11 : Constant  Value=0
  Constant12 : Constant  Value=5
  Constant5 : Constant  Value=0
  Delay{5..8} (4 alike) : UnitDelay  SampleTime=Tm
  Equal : RelationalOperator  Operator===
  Equal1 : RelationalOperator  Operator===
  Equal2 : RelationalOperator  Operator===
  Equal3 : RelationalOperator  Operator=<=
  Greater : RelationalOperator  Operator=>
  Greater2 : RelationalOperator  Operator=<
  Greater3 : RelationalOperator  Operator=<
  Product : Product  Inputs=*/  InputSameDT=on  SaturateOnIntegerOverflow=on  OutDataTypeStr=Inherit: Same as first input
  Product1 : Product  InputSameDT=on  SaturateOnIntegerOverflow=on  OutDataTypeStr=Inherit: Same as first input
  Product2 : Product  Inputs=/*  InputSameDT=on  SaturateOnIntegerOverflow=on  OutDataTypeStr=Inherit: Same as first input
  Smaller : RelationalOperator  Operator=<
  Smaller1 : RelationalOperator  Operator=>
  Smaller2 : RelationalOperator  Operator=>
  Smaller3 : RelationalOperator  Operator=>
  Sum6 : Sum  Inputs=|+-  InputSameDT=on  SaturateOnIntegerOverflow=on  OutDataTypeStr=Inherit: Same as first input
  Switch{4..8} (5 alike) : Switch  Threshold=0.5
  Tm{,1..3} (4 alike) : Constant  Value=Tm
  adelay2 : Subsystem
  adelay3 : Subsystem
  adelay4 : Subsystem
  adelay5 : Subsystem
  adelay6 : Subsystem
  and : Logic
  and1 : Logic
  and2 : Logic
  deltay : Subsystem
  pi : Constant  Value=pi
  three : Constant  Value=3
  uno : Constant
  xor : Logic  Operator=XOR
  zero{,1..5,8} (7 alike) : Constant  Value=0
  Tu : Outport
  a : Outport  Port=2
  D : Outport  Port=3
  Ku : Outport  Port=4
  sw : Outport  Port=5
  wires:
  y/1 -> Greater/1, Delay5/1, Greater2/1, Delay7/1, Equal2/1, Switch6/1
  Delay5/1 -> Smaller/1
  Greater/1 -> and2/1
  Smaller/1 -> and2/2
  Constant5/1 -> Greater/2, Smaller/2
  zero5/1 -> Switch4/3
  Switch4/1 -> adelay3/1(In1)
  zero/1 -> Switch6/3
  Tm/1 -> Switch4/1
  Delay7/1 -> Smaller1/1
  Greater2/1 -> and1/1
  Smaller1/1 -> and1/2
  Constant11/1 -> Greater2/2, Smaller1/2
  Constant12/1 -> Equal1/1
  deltay/1(Out1) -> Product/1
  Tm1/1 -> Product/2
  Delay6/1 -> Smaller2/1
  Greater3/1 -> and/1
  Smaller2/1 -> and/2
  zero1/1 -> Greater3/2, Smaller2/2
  Delay8/1 -> Switch5/1
  Switch6/1 -> deltay/1(In1), Delay8/1
  and/1 -> Switch5/2
  Product/1 -> Greater3/1, Delay6/1
  zero2/1 -> Switch5/3
  Equal1/1 -> Switch6/2
  Switch5/1 -> adelay5/1(In1)
  zero3/1 -> Equal2/2
  Equal2/1 -> Switch7/2
  Tm2/1 -> Switch7/1
  zero4/1 -> Switch7/3
  Tm3/1 -> Sum6/2
  adelay6/1(Out1) -> Sum6/1
  Switch7/1 -> adelay6/1(In1)
  zero8/1 -> Smaller3/2
  Smaller3/1 -> Switch8/2
  uno/1 -> Switch8/3
  Product1/1 -> Product2/1
  4pi/1 -> Product2/2
  pi/1 -> Product1/2
  Switch8/1 -> Product1/1
  three/1 -> Equal/2, Equal3/2
  adelay2/1(Out1) -> Equal/1, Equal3/1
  and2/1 -> adelay2/1(In1), xor/1
  xor/1 -> adelay4/1(In1)
  adelay3/1(Out1) -> Tu/1
  adelay5/1(Out1) -> a/1, Switch8/1, Smaller3/1
  Sum6/1 -> D/1
  Product2/1 -> Ku/1
  Equal3/1 -> sw/1
  Equal/1 -> Switch4/2
  adelay4/1(Out1) -> Equal1/2
  and1/1 -> xor/2

== system autotun2_1stor_mod/delay ==
  In1 : Inport
  Sum9 : Sum  Inputs=|+-  InputSameDT=on  SaturateOnIntegerOverflow=on  OutDataTypeStr=Inherit: Same as first input
  Unit Delay5 : UnitDelay  SampleTime=Tm
  Out1 : Outport
  wires:
  In1/1 -> Sum9/1, Unit Delay5/1
  Unit Delay5/1 -> Sum9/2
  Sum9/1 -> Out1/1

== system autotun2_1stor_mod/delay1 ==
  In1 : Inport
  Sum9 : Sum  Inputs=|+-  InputSameDT=on  SaturateOnIntegerOverflow=on  OutDataTypeStr=Inherit: Same as first input
  Unit Delay5 : UnitDelay  SampleTime=Tm
  Out1 : Outport
  wires:
  In1/1 -> Sum9/1, Unit Delay5/1
  Unit Delay5/1 -> Sum9/2
  Sum9/1 -> Out1/1

== system autotun2_1stor_mod/Derivative/delay2 ==
  In1 : Inport
  Sum9 : Sum  Inputs=|+-  InputSameDT=on  SaturateOnIntegerOverflow=on  OutDataTypeStr=Inherit: Same as first input
  Unit Delay5 : UnitDelay  SampleTime=Tm
  Out1 : Outport
  wires:
  Sum9/1 -> Out1/1
  In1/1 -> Sum9/1, Unit Delay5/1
  Unit Delay5/1 -> Sum9/2

== system autotun2_1stor_mod/Derivative1/delay2 ==
  In1 : Inport
  Sum9 : Sum  Inputs=|+-  InputSameDT=on  SaturateOnIntegerOverflow=on  OutDataTypeStr=Inherit: Same as first input
  Unit Delay5 : UnitDelay  SampleTime=Tm
  Out1 : Outport
  wires:
  Sum9/1 -> Out1/1
  In1/1 -> Sum9/1, Unit Delay5/1
  Unit Delay5/1 -> Sum9/2

== system autotun2_1stor_mod/Integral/adelay1 ==
  In1 : Inport
  Sum9 : Sum  Inputs=|++  InputSameDT=on  SaturateOnIntegerOverflow=on  OutDataTypeStr=Inherit: Same as first input
  Unit Delay6 : UnitDelay  SampleTime=Tm
  Out1 : Outport
  wires:
  In1/1 -> Sum9/1
  Unit Delay6/1 -> Sum9/2
  Sum9/1 -> Out1/1, Unit Delay6/1

== system autotun2_1stor_mod/Integral1/adelay1 ==
  In1 : Inport
  Sum9 : Sum  Inputs=|++  InputSameDT=on  SaturateOnIntegerOverflow=on  OutDataTypeStr=Inherit: Same as first input
  Unit Delay6 : UnitDelay  SampleTime=Tm
  Out1 : Outport
  wires:
  In1/1 -> Sum9/1
  Unit Delay6/1 -> Sum9/2
  Sum9/1 -> Out1/1, Unit Delay6/1

== system autotun2_1stor_mod/auto-tuner/adelay2 ==
  In1 : Inport
  Sum9 : Sum  Inputs=|++  InputSameDT=on  SaturateOnIntegerOverflow=on  OutDataTypeStr=Inherit: Same as first input
  Unit Delay6 : UnitDelay  SampleTime=Tm
  Out1 : Outport
  wires:
  In1/1 -> Sum9/1
  Unit Delay6/1 -> Sum9/2
  Sum9/1 -> Out1/1, Unit Delay6/1

== system autotun2_1stor_mod/auto-tuner/adelay3 ==
  In1 : Inport
  Sum9 : Sum  Inputs=|++  InputSameDT=on  SaturateOnIntegerOverflow=on  OutDataTypeStr=Inherit: Same as first input
  Unit Delay6 : UnitDelay  SampleTime=Tm
  Out1 : Outport
  wires:
  In1/1 -> Sum9/1
  Unit Delay6/1 -> Sum9/2
  Sum9/1 -> Out1/1, Unit Delay6/1

== system autotun2_1stor_mod/auto-tuner/adelay4 ==
  In1 : Inport
  Sum9 : Sum  Inputs=|++  InputSameDT=on  SaturateOnIntegerOverflow=on  OutDataTypeStr=Inherit: Same as first input
  Unit Delay6 : UnitDelay  SampleTime=Tm
  Out1 : Outport
  wires:
  In1/1 -> Sum9/1
  Unit Delay6/1 -> Sum9/2
  Sum9/1 -> Out1/1, Unit Delay6/1

== system autotun2_1stor_mod/auto-tuner/adelay5 ==
  In1 : Inport
  Sum9 : Sum  Inputs=|++  InputSameDT=on  SaturateOnIntegerOverflow=on  OutDataTypeStr=Inherit: Same as first input
  Unit Delay6 : UnitDelay  SampleTime=Tm
  Out1 : Outport
  wires:
  In1/1 -> Sum9/1
  Unit Delay6/1 -> Sum9/2
  Sum9/1 -> Out1/1, Unit Delay6/1

== system autotun2_1stor_mod/auto-tuner/adelay6 ==
  In1 : Inport
  Sum9 : Sum  Inputs=|++  InputSameDT=on  SaturateOnIntegerOverflow=on  OutDataTypeStr=Inherit: Same as first input
  Unit Delay6 : UnitDelay  SampleTime=Tm
  Out1 : Outport
  wires:
  In1/1 -> Sum9/1
  Unit Delay6/1 -> Sum9/2
  Sum9/1 -> Out1/1, Unit Delay6/1

== system autotun2_1stor_mod/auto-tuner/deltay ==
  In1 : Inport
  Sum9 : Sum  Inputs=|+-  InputSameDT=on  SaturateOnIntegerOverflow=on  OutDataTypeStr=Inherit: Same as first input
  Unit Delay5 : UnitDelay  SampleTime=Tm
  Out1 : Outport
  wires:
  In1/1 -> Sum9/1, Unit Delay5/1
  Unit Delay5/1 -> Sum9/2
  Sum9/1 -> Out1/1
